simulink model "HILModelFull"  (Simulink 6.6)
settings: Solver=ode4  StartTime=0.0  StopTime=inf  FixedStep=SampleT  RelTol=1e-3
InitFcn:
  | clc
  | Taxi_Var_new
  | failures
  | insInit
  | piccolo_init
values from neighbouring files (symbols this model uses):
  A1 = 0    [Taxi_Var.m]
  Apolar = 0.0899    [Taxi_Var.m]
  CD0 = 0.0219    [Taxi_Var.m]
  chord = S/span    (= 0.384036716878)    [Taxi_Var.m]
  CL0 = 0.1857    [Taxi_Var.m]
  CLa = 4.6206    [Taxi_Var.m]
  CLa_dot = 1.93    [Taxi_Var.m]
  Clb = -0.0043    [Taxi_Var.m]
  ClDa = 0.1695    [Taxi_Var.m]
  CLDe = 0.4032    [Taxi_Var.m]
  CLDf = 0.047    [Taxi_Var.m]
  ClDr = 0.0003    [Taxi_Var.m]
  Clp = -0.4425    [Taxi_Var.m]
  CLq = 8.7465    [Taxi_Var.m]
  Clr = 0.0675    [Taxi_Var.m]
  Cm0 = -0.0902    [Taxi_Var.m]
  Cma = -1.3995    [Taxi_Var.m]
  CmDe = -0.9493    [Taxi_Var.m]
  CmDf = -.021    (= -0.021)    [Taxi_Var.m]
  Cmq = -10.8760    (= -10.876)    [Taxi_Var.m]
  Cnb = 0.0281    [Taxi_Var.m]
  CnDa = -0.0031    [Taxi_Var.m]
  CnDr = -0.0882    [Taxi_Var.m]
  Cnp = -0.0695    [Taxi_Var.m]
  Cnr = -0.1045    [Taxi_Var.m]
  CYb = -0.1999    [Taxi_Var.m]
  CYDr = 0.0192    [Taxi_Var.m]
  damax = 25*deg2rad    (= 0.436332312999)    [Taxi_Var.m]
  damin = -25*deg2rad    (= -0.436332312999)    [Taxi_Var.m]
  datrim = 0*deg2rad    (= 0)    [Taxi_Var.m]
  demax = 15*deg2rad    (= 0.261799387799)    [Taxi_Var.m]
  demin = -15*deg2rad    (= -0.261799387799)    [Taxi_Var.m]
  detrim = -2.4137*deg2rad    (= -0.0421270121554)    [Taxi_Var.m]
  dfland = 30*deg2rad    (= 0.523598775598)    [Taxi_Var.m]
  dfmax = 30*deg2rad    (= 0.523598775598)    [Taxi_Var.m]
  dfmin = 0*deg2rad    (= 0)    [Taxi_Var.m]
  drmax = 25*deg2rad    (= 0.436332312999)    [Taxi_Var.m]
  drmin = -25*deg2rad    (= -0.436332312999)    [Taxi_Var.m]
  drtrim = 0*deg2rad    (= 0)    [Taxi_Var.m]
  dtmax = 1    [Taxi_Var.m]
  dtmin = 0    [Taxi_Var.m]
  dttrim = 0.0725    [Taxi_Var.m]
  Euler_0 = [0; 0; 45]'*pi/180    [Taxi_Var.m]    (also in hilInit.m = [0; 0; 0*pi/180]')
  HIL_K = 3    [hilInit.m]    (also in insInit.m)
  ISA_g = 9.815    [Taxi_Var.m]
  ISA_hmax = 2000    [Taxi_Var.m]
  ISA_lapse = .0065    (= 0.0065)    [Taxi_Var.m]
  ISA_P0 = 101325    [Taxi_Var.m]
  ISA_R = 287    [Taxi_Var.m]
  ISA_rho0 = 1.225    [Taxi_Var.m]
  ISA_T0 = 289    [Taxi_Var.m]
  Ixx = 3.689084    [Taxi_Var.m]
  Iyy = 7.43789    [Taxi_Var.m]
  Izz = 10.22202    [Taxi_Var.m]
  mass = 22.5    [Taxi_Var.m]
  MinThK = 0.075    [Taxi_Var.m]
  Pos_0 = [0; 0; 1000]'    [Taxi_Var.m]    (also in hilInit.m = [500; 750; 350]')
  PQR_0 = [0; 0; 0]'    [Taxi_Var.m]
  span = 2.3368    [Taxi_Var.m]
  TFact = 0.4    [Taxi_Var.m]
  ThK = 2.18    [Taxi_Var.m]
  Vb_0 = [35; 0; 0]'    [Taxi_Var.m]
undefined symbols (not defined in the file or in its folder): clock, Earth, IdxCmdOrbitRadius, IdxCmdOrbitSense, IdxCmdWp1Alt, IdxCmdWp1Lat, IdxCmdWp1Lon, IdxCmdWp2Alt, IdxCmdWp2Lat, IdxCmdWp2Lon, IdxEstimReserved1, IdxEstimWEast, IdxEstimWNorth, IdxGainsAltD, IdxGainsAltI, IdxGainsAltP, IdxGainsPdynD, IdxGainsPdynI, IdxGainsPdynP, IdxGainsPitchD, IdxGainsPitchI, IdxGainsPitchP, IdxGainsRollD, IdxGainsRollI, IdxGainsRollP, IdxGainsSlopeElevatorD, IdxGainsSlopeElevatorP, IdxGainsTrackConv, IdxGainsTrackD, IdxGainsTrackI, IdxGainsTrackP, IdxGainsTurnD, IdxGainsTurnI, IdxGainsTurnP, IdxGainsYawD, IdxGainsYawI, IdxGainsYawP, IdxLimitsAileronMax, IdxLimitsAileronMin, IdxLimitsBankMax, IdxLimitsBankMin, IdxLimitsElevatorMax, IdxLimitsElevatorMin, IdxLimitsFlapMax, IdxLimitsFlapMin, IdxLimitsPdynMax, IdxLimitsPdynMin, IdxLimitsRudderMax, IdxLimitsRudderMin, IdxLimitsThrottleMax, IdxLimitsThrottleMin, IdxSensorsAlt, IdxSensorsLat, IdxSensorsLon, IdxSensorsVDown, IdxSensorsVEast, IdxSensorsVNorth, IdxStatesGlobal, IdxStatesManual, IdxStatesMode ... (+3)
libraries: piccolo_library x60, simulink x33, xpclib x8, aerolibasang x5, aerolibconvert2 x5, aerolibtransform2 x2, aerolibnav x2, aerolibatmos2 x1, dspmtrx3 x1
(part 2 of 4)

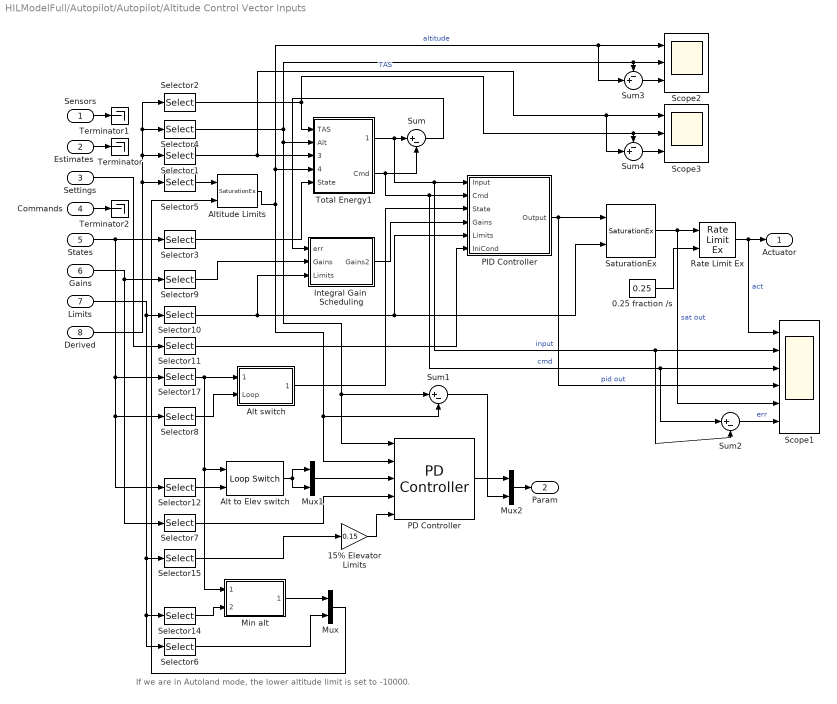
== system HILModelFull/Autopilot/Autopilot/Altitude Control Vector Inputs ==
  note: If we are in Autoland mode, the lower altitude limit is set to -10000.
  Sensors : Inport  PortDimensions=SizeSensors
  Estimates : Inport  Port=2  PortDimensions=SizeEstim
  Settings : Inport  Port=3  PortDimensions=SizeSet
  Commands : Inport  Port=4  PortDimensions=SizeCmd
  States : Inport  Port=5  PortDimensions=SizeStates
  Gains : Inport  Port=6  PortDimensions=SizeGains
  Limits : Inport  Port=7  PortDimensions=SizeLimits
  Derived : Inport  Port=8  PortDimensions=SizeDrv
  0.25 fraction /s : Constant  Value=0.25
  15% Elevator Limits : Gain  Gain=0.15  SaturateOnIntegerOverflow=on
  Alt switch : Subsystem  AncestorBlock=piccolo_library/Logic/DynP-Alt-Turn switch
  Alt to Elev switch : piccolo_library/Logic/Loop Switch  SystemSampleTime=-1
  Altitude Limits : piccolo_library/Nonlinear/SaturationEx  SystemSampleTime=-1
  Integral Gain  Scheduling : Subsystem
  Min alt : Subsystem
      mask Type: Loop Switch
      mask Description:
      | Select whether this individual loop is enabled or disabled.  This is done based on the specific
      | loop enable state, and the global flag.  In auto or manual steering the loop is on.  In Manual
      | or AutoLaunch the loop should be off.
  Mux : Mux  Inputs=2
  Mux1 : Mux  Inputs=2
  Mux2 : Mux  Inputs=2
  PD Controller : piccolo_library/Controllers/PD Controller  SystemSampleTime=-1  tsamp=tsamp  tdelay=0.5
  PID Controller : Subsystem  AncestorBlock=piccolo_library/Controllers/PID Controller  mask(PID Controller){tsamp=tsamp, tdelay=1}
      mask prompts: tsamp "Sample time:"; tdelay "Time derivative delay:"
      mask help: Generic PID (proportional, integral, derivative) controller with a single input and a single output.
  Rate Limit Ex : piccolo_library/Nonlinear/Rate Limit Ex  SystemSampleTime=-1  T=tsamp
  SaturationEx : piccolo_library/Nonlinear/SaturationEx  SystemSampleTime=-1
  Scope1 : Scope  NumInputPorts=6
      settings: YMin=0.120001~972.462~972.462~0.120001~0.120001~5.25e-006  YMax=0.120001~972.462~972.462~0.120001~0.120001~7e-006
  Scope2 : Scope  NumInputPorts=3
      settings: YMin=855~900.05~-0.475  YMax=945~900.475~-0.05  SaveName=ScopeData14
  Scope3 : Scope  NumInputPorts=3
      settings: YMin=35.0006~35~-0.035  YMax=35.0008~35.035~3.46945e-018  SaveName=ScopeData17
  Selector1 : Selector  IndexOptions=Index vector (dialog)  Indices=IdxDrvTASCmdNom  OutputSizes=1  InputPortWidth=SizeDrv
  Selector10 : Selector  IndexOptions=Index vector (dialog)  Indices=[IdxLimitsThrottleMin IdxLimitsThrottleMax]  OutputSizes=1  InputPortWidth=SizeLimits
  Selector11 : Selector  IndexOptions=Index vector (dialog)  Indices=IdxSetThrottleTrim  OutputSizes=1  InputPortWidth=SizeSet
  Selector12 : Selector  IndexOptions=Index vector (dialog)  Indices=IdxStatesAltToElev  OutputSizes=1  InputPortWidth=SizeStates
  Selector14 : Selector  IndexOptions=Index vector (dialog)  Indices=IdxLimitsAltMin  OutputSizes=1  InputPortWidth=SizeLimits
  Selector15 : Selector  IndexOptions=Index vector (dialog)  Indices=[IdxLimitsElevatorMin IdxLimitsElevatorMax]  OutputSizes=1  InputPortWidth=SizeLimits
  Selector17 : Selector  IndexOptions=Index vector (dialog)  Indices=[IdxStatesGlobal IdxStatesMode IdxStatesManual]  OutputSizes=1  InputPortWidth=SizeStates
  Selector2 : Selector  IndexOptions=Index vector (dialog)  Indices=IdxDrvTAS  OutputSizes=1  InputPortWidth=SizeDrv
  Selector3 : Selector  IndexOptions=Index vector (dialog)  Indices=IdxStatesPdyn  OutputSizes=1  InputPortWidth=SizeStates
  Selector4 : Selector  IndexOptions=Index vector (dialog)  Indices=IdxDrvBaroAlt  OutputSizes=1  InputPortWidth=SizeDrv
  Selector5 : Selector  IndexOptions=Index vector (dialog)  Indices=IdxDrvAltCmd  OutputSizes=1  InputPortWidth=SizeDrv
  Selector6 : Selector  IndexOptions=Index vector (dialog)  Indices=IdxLimitsAltMax  OutputSizes=1  InputPortWidth=SizeLimits
  Selector7 : Selector  IndexOptions=Index vector (dialog)  Indices=[IdxGainsSlopeElevatorP IdxGainsSlopeElevatorD]  OutputSizes=1  InputPortWidth=SizeGains
  Selector8 : Selector  IndexOptions=Index vector (dialog)  Indices=IdxStatesAlt  OutputSizes=1  InputPortWidth=SizeStates
  Selector9 : Selector  IndexOptions=Index vector (dialog)  Indices=[IdxGainsAltP IdxGainsAltI IdxGainsAltD]  OutputSizes=1  InputPortWidth=SizeGains
  Sum : Sum  Inputs=|+-  SaturateOnIntegerOverflow=on
  Sum1 : Sum  Inputs=|+-  SaturateOnIntegerOverflow=on
  Sum2 : Sum  Inputs=|+-  SaturateOnIntegerOverflow=on
  Sum3 : Sum  Inputs=-+|  SaturateOnIntegerOverflow=on
  Sum4 : Sum  Inputs=-+|  SaturateOnIntegerOverflow=on
  Terminator : Terminator
  Terminator1 : Terminator
  Terminator2 : Terminator
  Total Energy1 : Subsystem
      mask Type: Total Energy
      mask Description: Compute the total energy state and command as a sum of kinetic and potential energies, in units of altitude
  Actuator : Outport  OutDataType=fixdt(1,16,0)  OutScaling=[]
  Param : Outport  Port=2  OutDataType=fixdt(1,16,0)  OutScaling=[]
  wires:
  Total Energy1/2(Cmd) -> Sum/2, PID Controller/2(Cmd), Scope1/3, Sum2/1  "cmd"
  Total Energy1/1(Energy) -> Sum/1, PID Controller/1(Input), Scope1/2, Sum2/2  "input"
  Selector3/1 -> Total Energy1/5(State)
  Selector1/1 -> Total Energy1/3(TASCmd), Scope3/1, Sum4/2  "TAS"
  PD Controller/1 -> Mux2/1
  Mux2/1 -> Param/1
  Sum1/1 -> Mux2/2
  Commands/1 -> Terminator2/1
  States/1 -> Selector3/1, Selector12/1, Selector8/1, Selector17/1
  Sum/1 -> Integral Gain  Scheduling/1(err)
  Selector7/1 -> PD Controller/4
  Mux1/1 -> PD Controller/3
  Alt to Elev switch/1 -> Mux1/2, Mux1/1
  Selector15/1 -> 15% Elevator Limits/1
  15% Elevator Limits/1 -> PD Controller/5
  Selector9/1 -> Integral Gain  Scheduling/2(Gains)
  Integral Gain  Scheduling/1(Gains2) -> PID Controller/4(Gains)
  Mux/1 -> Altitude Limits/2
  Selector6/1 -> Mux/2
  Min alt/1(MinAltOut) -> Mux/1
  Selector14/1 -> Min alt/2(MinAlt)
  Selector12/1 -> Alt to Elev switch/2
  PID Controller/1(Output) -> SaturationEx/1, Scope1/4  "pid out"
  Derived/1 -> Selector1/1, Selector4/1, Selector2/1, Selector5/1
  Selector5/1 -> Altitude Limits/1
  Altitude Limits/1 -> Sum1/2, PD Controller/2, Total Energy1/4(AltCmd), Scope2/1, Sum3/2  "altitude"
  Selector4/1 -> Total Energy1/2(Alt), Sum1/1, PD Controller/1, Scope2/2, Sum3/1
  Selector2/1 -> Total Energy1/1(TAS), Scope3/2, Sum4/1
  Sensors/1 -> Terminator1/1
  Rate Limit Ex/1 -> Actuator/1, Scope1/1  "act"
  0.25 fraction /s/1 -> Rate Limit Ex/2
  SaturationEx/1 -> Rate Limit Ex/1, Scope1/5  "sat out"
  Selector10/1 -> Integral Gain  Scheduling/3(Limits), SaturationEx/2, PID Controller/5(Limits)
  Limits/1 -> Selector15/1, Selector6/1, Selector14/1, Selector10/1
  Gains/1 -> Selector7/1, Selector9/1
  Selector11/1 -> PID Controller/6(IniCond)
  Settings/1 -> Selector11/1
  Selector17/1 -> Alt switch/1(Globals), Min alt/1(Globals), Alt to Elev switch/1
  Selector8/1 -> Alt switch/2(Loop)
  Alt switch/1(TriOut) -> PID Controller/3(State)
  Estimates/1 -> Terminator/1
  Sum2/1 -> Scope1/6  "err"
  Sum3/1 -> Scope2/3
  Sum4/1 -> Scope3/3

== system HILModelFull/Autopilot/Autopilot/Flap Control Vector Inputs ==
  Sensors : Inport  PortDimensions=SizeSensors
  Estimates : Inport  Port=2  PortDimensions=SizeEstim
  Settings : Inport  Port=3  PortDimensions=SizeSet
  Commands : Inport  Port=4  PortDimensions=SizeCmd
  States : Inport  Port=5  PortDimensions=SizeStates
  Gains : Inport  Port=6  PortDimensions=SizeGains
  Limits : Inport  Port=7  PortDimensions=SizeLimits
  Derived : Inport  Port=8  PortDimensions=SizeDrv
  5 deg/s : Constant  Value=10*pi/180
  Direct Flap Control : Selector  IndexOptions=Index vector (dialog)  Indices=IdxCmdFlap  OutputSizes=1  InputPortWidth=SizeCmd
  Flap Loop Switch : piccolo_library/Logic/Loop Switch  SystemSampleTime=-1
  Landing Flap : Selector  IndexOptions=Index vector (dialog)  Indices=IdxSetLandingFlap  OutputSizes=1  InputPortWidth=SizeSet
  Rate Limit Ex : piccolo_library/Nonlinear/Rate Limit Ex  SystemSampleTime=-1  T=tsamp
  SaturationEx : piccolo_library/Nonlinear/SaturationEx  SystemSampleTime=-1
  Selector1 : Selector  IndexOptions=Index vector (dialog)  Indices=[IdxStatesGlobal IdxStatesMode IdxStatesManual]  OutputSizes=1  InputPortWidth=SizeStates
  Selector10 : Selector  IndexOptions=Index vector (dialog)  Indices=[IdxLimitsFlapMin IdxLimitsFlapMax]  OutputSizes=1  InputPortWidth=SizeLimits
  Selector12 : Selector  IndexOptions=Index vector (dialog)  Indices=IdxStatesSlope  OutputSizes=1  InputPortWidth=SizeStates
  Selector2 : Selector  IndexOptions=Index vector (dialog)  Indices=IdxStatesFlap  OutputSizes=1  InputPortWidth=SizeStates
  Switch : Switch  Threshold=0.5  SaturateOnIntegerOverflow=on
  Switch1 : Switch  Threshold=0.5  SaturateOnIntegerOverflow=on
  Terminator{1..4} (4 alike) : Terminator
  Zero : Constant  Value=0
  Actuator : Outport  OutDataType=fixdt(1,16,0)  OutScaling=[]
  wires:
  Sensors/1 -> Terminator1/1
  Selector10/1 -> SaturationEx/2
  Selector12/1 -> Switch/2
  Direct Flap Control/1 -> Switch/3
  Landing Flap/1 -> Switch/1
  Estimates/1 -> Terminator2/1
  Gains/1 -> Terminator3/1
  Derived/1 -> Terminator4/1
  Settings/1 -> Landing Flap/1
  Commands/1 -> Direct Flap Control/1
  States/1 -> Selector12/1, Selector2/1, Selector1/1
  Limits/1 -> Selector10/1
  Switch/1 -> Switch1/1
  Flap Loop Switch/1 -> Switch1/2
  Switch1/1 -> SaturationEx/1
  Selector1/1 -> Flap Loop Switch/1
  Selector2/1 -> Flap Loop Switch/2
  Zero/1 -> Switch1/3
  SaturationEx/1 -> Rate Limit Ex/1
  Rate Limit Ex/1 -> Actuator/1
  5 deg/s/1 -> Rate Limit Ex/2

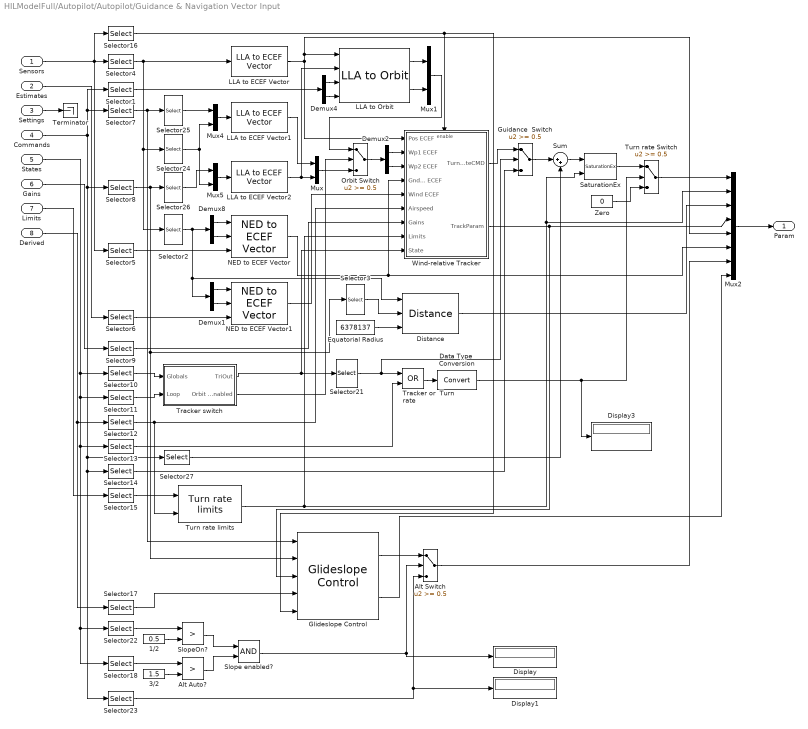
== system HILModelFull/Autopilot/Autopilot/Guidance & Navigation Vector Input ==
  Sensors : Inport  PortDimensions=SizeSensors
  Estimates : Inport  Port=2  PortDimensions=SizeEstim
  Settings : Inport  Port=3  PortDimensions=SizeSet
  Commands : Inport  Port=4  PortDimensions=SizeCmd
  States : Inport  Port=5  PortDimensions=SizeStates
  Gains : Inport  Port=6  PortDimensions=SizeGains
  Limits : Inport  Port=7  PortDimensions=SizeLimits
  Derived : Inport  Port=8  PortDimensions=SizeDrv
  1/2 : Constant  Value=0.5
  3/2 : Constant  Value=1.5
  Alt Auto? : RelationalOperator  Operator=>
  Alt Switch : Switch  Threshold=0.5  SaturateOnIntegerOverflow=on
  Data Type  Conversion : DataTypeConversion  OutDataTypeMode=double  OutDataType=fixdt(1,16,0)  OutScaling=[]  SaturateOnIntegerOverflow=on  RndMeth=Zero
  Demux{1..2,4,8} (4 alike) : Demux  Outputs=2
  Display : Display
  Display1 : Display
  Display3 : Display
  Distance : piccolo_library/Transformations/Distance  SystemSampleTime=-1
  Equatorial Radius : Constant  Value=6378137
  Glideslope Control : piccolo_library/Controllers/Guidance/Glideslope Control  SystemSampleTime=-1  tsamp=tsamp  aptsamp=aptsamp
  Guidance  Switch : Switch  Threshold=0.5  SaturateOnIntegerOverflow=on
  LLA to ECEF Vector : piccolo_library/Transformations/LLA to ECEF Vector  SystemSampleTime=-1
  LLA to ECEF Vector1 : piccolo_library/Transformations/LLA to ECEF Vector  SystemSampleTime=-1
  LLA to ECEF Vector2 : piccolo_library/Transformations/LLA to ECEF Vector  SystemSampleTime=-1
  LLA to Orbit : piccolo_library/Controllers/Guidance/LLA to Orbit  SystemSampleTime=-1
  Mux{,1,4..5} (4 alike) : Mux  Inputs=2
  Mux2 : Mux  Inputs=[1 2 1 5 3 3 1 3]
  NED to ECEF Vector : piccolo_library/Transformations/NED to ECEF Vector  SystemSampleTime=-1
  NED to ECEF Vector1 : piccolo_library/Transformations/NED to ECEF Vector  SystemSampleTime=-1
  Orbit Switch : Switch  Threshold=0.5  SaturateOnIntegerOverflow=on
  SaturationEx : piccolo_library/Nonlinear/SaturationEx  SystemSampleTime=-1
  Selector1 : Selector  IndexOptions=Index vector (dialog)  Indices=[IdxCmdOrbitRadius IdxCmdOrbitSense]  OutputSizes=1  InputPortWidth=SizeCmd
  Selector10 : Selector  IndexOptions=Index vector (dialog)  Indices=[IdxStatesGlobal IdxStatesMode IdxStatesManual]  OutputSizes=1  InputPortWidth=SizeStates
  Selector11 : Selector  IndexOptions=Index vector (dialog)  Indices=IdxStatesTracker  OutputSizes=1  InputPortWidth=SizeStates
  Selector12 : Selector  IndexOptions=Index vector (dialog)  Indices=IdxDrvTAS  OutputSizes=1  InputPortWidth=SizeDrv
  Selector13 : Selector  IndexOptions=Index vector (dialog)  Indices=IdxStatesTurnRate  OutputSizes=1  InputPortWidth=SizeStates
  Selector14 : Selector  IndexOptions=Index vector (dialog)  Indices=IdxCmdTurnRate  OutputSizes=1  InputPortWidth=SizeCmd
  Selector15 : Selector  IndexOptions=Index vector (dialog)  Indices=[IdxLimitsBankMin IdxLimitsBankMax]  OutputSizes=1  InputPortWidth=SizeLimits
  Selector16 : Selector  IndexOptions=Index vector (dialog)  Indices=IdxSensorsGPSNew  OutputSizes=1  InputPortWidth=SizeSensors
  Selector17 : Selector  IndexOptions=Index vector (dialog)  Indices=IdxDrvBaroAlt  OutputSizes=1  InputPortWidth=SizeDrv
  Selector18 : Selector  IndexOptions=Index vector (dialog)  Indices=IdxStatesAlt  OutputSizes=1  InputPortWidth=SizeStates
  Selector{2..3,25..26} (4 alike) : Selector  IndexOptions=Index vector (dialog)  Indices=[1 2]  OutputSizes=1  InputPortWidth=3
  Selector21 : Selector  IndexOptions=Index vector (dialog)  Indices=2  OutputSizes=1  InputPortWidth=3
  Selector22 : Selector  IndexOptions=Index vector (dialog)  Indices=IdxStatesSlope  OutputSizes=1  InputPortWidth=SizeStates
  Selector23 : Selector  IndexOptions=Index vector (dialog)  Indices=IdxCmdAlt  OutputSizes=1  InputPortWidth=SizeCmd
  Selector24 : Selector  IndexOptions=Index vector (dialog)  Indices=3  OutputSizes=1  InputPortWidth=3
  Selector27 : Selector  IndexOptions=Index vector (dialog)  Indices=IdxCmdTurnRateShift  OutputSizes=1  InputPortWidth=SizeCmd
  Selector4 : Selector  IndexOptions=Index vector (dialog)  Indices=[IdxSensorsLat IdxSensorsLon IdxSensorsAlt]  OutputSizes=1  InputPortWidth=SizeSensors
  Selector5 : Selector  IndexOptions=Index vector (dialog)  Indices=[IdxSensorsVNorth IdxSensorsVEast IdxSensorsVDown]  OutputSizes=1  InputPortWidth=SizeSensors
  Selector6 : Selector  IndexOptions=Index vector (dialog)  Indices=[IdxEstimWNorth IdxEstimWEast IdxEstimReserved1]  OutputSizes=1  InputPortWidth=SizeEstim
  Selector7 : Selector  IndexOptions=Index vector (dialog)  Indices=[IdxCmdWp1Lat IdxCmdWp1Lon IdxCmdWp1Alt]  OutputSizes=1  InputPortWidth=SizeCmd
  Selector8 : Selector  IndexOptions=Index vector (dialog)  Indices=[IdxCmdWp2Lat IdxCmdWp2Lon IdxCmdWp2Alt]  OutputSizes=1  InputPortWidth=SizeCmd
  Selector9 : Selector  IndexOptions=Index vector (dialog)  Indices=[IdxGainsTrackP IdxGainsTrackI IdxGainsTrackD IdxGainsTrackConv]  OutputSizes=1  InputPortWidth=SizeGains
  Slope enabled? : Logic  AllPortsSameDT=off
  SlopeOn? : RelationalOperator  Operator=>
  Sum : Sum  Inputs=|++  SaturateOnIntegerOverflow=on
  Terminator : Terminator
  Tracker or  Turn rate : Logic  Operator=OR  AllPortsSameDT=off
  Tracker switch : Subsystem  AncestorBlock=piccolo_library/Logic/Tracker switch
  Turn rate Switch : Switch  Threshold=0.5  SaturateOnIntegerOverflow=on
  Turn rate limits : piccolo_library/Flight Mechanics/Turn rate limits  SystemSampleTime=-1
  Wind-relative Tracker : Subsystem  AncestorBlock=piccolo_library/Controllers/Guidance/Wind-relative Tracker  mask(Wind-relative Tracker){tsamp=tsamp}
      mask prompts: tsamp "Sample time:"
      mask help: A lateral track control law that takes into account the wind speed.
  Zero : Constant  Value=0
  Param : Outport  OutDataType=fixdt(1,16,0)  OutScaling=[]
  wires:
  Slope enabled?/1 -> Alt Switch/2, Display/1
  Alt Auto?/1 -> Slope enabled?/2
  SlopeOn?/1 -> Slope enabled?/1
  3/2/1 -> Alt Auto?/2
  Selector18/1 -> Alt Auto?/1
  Selector22/1 -> SlopeOn?/1
  1/2/1 -> SlopeOn?/2
  Selector21/1 -> Tracker or  Turn rate/1, Guidance  Switch/2
  Selector27/1 -> Sum/2
  Sum/1 -> SaturationEx/1
  Guidance  Switch/1 -> Sum/1
  Glideslope Control/2 -> Mux2/8
  Glideslope Control/1 -> Alt Switch/1
  Selector17/1 -> Glideslope Control/4
  Selector26/1 -> Mux5/1
  Selector7/1 -> Glideslope Control/1, Selector25/1
  Selector25/1 -> Mux4/1
  Selector24/1 -> Mux5/2, Mux4/2
  Mux5/1 -> LLA to ECEF Vector2/1
  Mux4/1 -> LLA to ECEF Vector1/1
  Alt Switch/1 -> Mux2/7
  Selector23/1 -> Alt Switch/3, Display1/1
  LLA to Orbit/2 -> Mux1/2
  LLA to Orbit/1 -> Mux1/1
  Selector1/1 -> Demux4/1
  Demux4/2 -> LLA to Orbit/4
  Demux4/1 -> LLA to Orbit/3
  Selector16/1 -> Glideslope Control/5, Wind-relative Tracker/Enable
  Settings/1 -> Terminator/1
  Data Type  Conversion/1 -> Turn rate Switch/2, Display3/1
  Wind-relative Tracker/2(TrackParam) -> Glideslope Control/3, Mux2/4
  Distance/1 -> Mux2/3
  Zero/1 -> Turn rate Switch/3
  SaturationEx/1 -> Turn rate Switch/1
  Tracker or  Turn rate/1 -> Data Type  Conversion/1
  Selector13/1 -> Tracker or  Turn rate/2
  Turn rate limits/1 -> Mux2/2, SaturationEx/2, Wind-relative Tracker/8(Limits)
  Limits/1 -> Selector15/1
  Selector15/1 -> Turn rate limits/1
  Selector14/1 -> Guidance  Switch/3
  Wind-relative Tracker/1(TurnRateCMD) -> Guidance  Switch/1
  Mux2/1 -> Param/1
  Tracker switch/1(TriOut) -> Wind-relative Tracker/9(State), Selector21/1
  Tracker switch/2(Orbit Enabled) -> Orbit Switch/2
  Selector11/1 -> Tracker switch/2(Loop)
  Selector10/1 -> Tracker switch/1(Globals)
  Derived/1 -> Selector17/1, Selector12/1
  States/1 -> Selector18/1, Selector22/1, Selector13/1, Selector11/1, Selector10/1
  Gains/1 -> Selector9/1
  Commands/1 -> Selector1/1, Selector7/1, Selector27/1, Selector23/1, Selector14/1, Selector8/1
  Selector8/1 -> Glideslope Control/2, Selector3/1, Selector26/1
  Estimates/1 -> Selector6/1
  Selector5/1 -> NED to ECEF Vector/3
  Sensors/1 -> Selector16/1, Selector5/1, Selector4/1
  Selector4/1 -> Selector2/1, Selector24/1, LLA to ECEF Vector/1
  Demux8/1 -> NED to ECEF Vector/1
  Demux8/2 -> NED to ECEF Vector/2
  Selector2/1 -> Demux8/1, Demux1/1, Distance/1
  Demux1/1 -> NED to ECEF Vector1/1
  Demux1/2 -> NED to ECEF Vector1/2
  Selector6/1 -> NED to ECEF Vector1/3
  LLA to ECEF Vector/1 -> LLA to Orbit/1, Mux2/5, Wind-relative Tracker/1(Pos ECEF)
  LLA to ECEF Vector2/1 -> LLA to Orbit/2, Mux/2
  Selector9/1 -> Wind-relative Tracker/7(Gains)
  LLA to ECEF Vector1/1 -> Mux/1
  Mux/1 -> Orbit Switch/3
  Mux1/1 -> Orbit Switch/1
  Demux2/1 -> Wind-relative Tracker/2(Wp1 ECEF)
  Demux2/2 -> Wind-relative Tracker/3(Wp2 ECEF)
  Orbit Switch/1 -> Demux2/1
  NED to ECEF Vector/1 -> Mux2/6, Wind-relative Tracker/4(Gndspd ECEF)
  NED to ECEF Vector1/1 -> Wind-relative Tracker/5(Wind ECEF)
  Selector12/1 -> Turn rate limits/2, Wind-relative Tracker/6(Airspeed)
  Equatorial Radius/1 -> Distance/3
  Selector3/1 -> Distance/2
  Turn rate Switch/1 -> Mux2/1

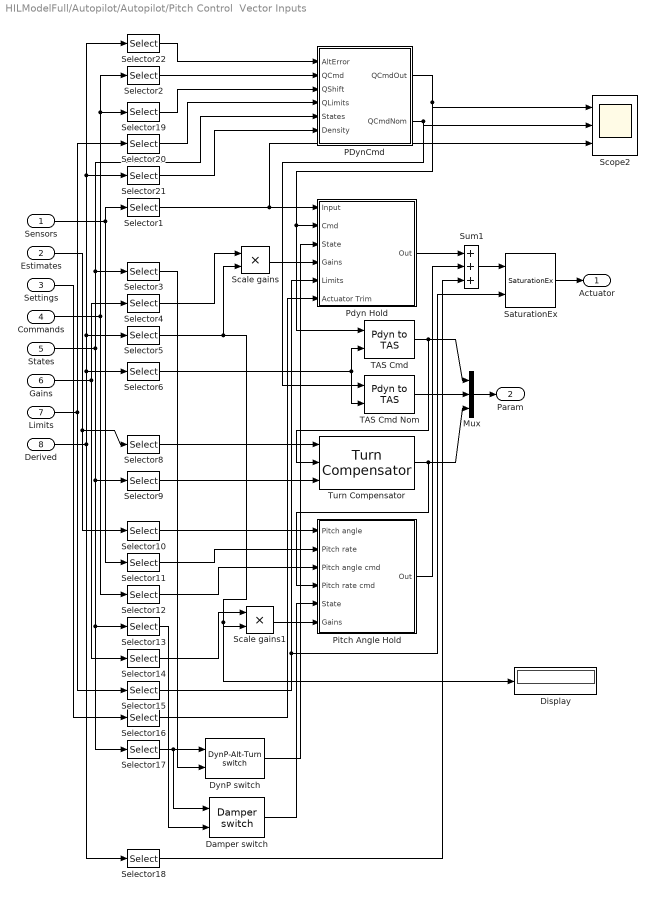
== system HILModelFull/Autopilot/Autopilot/Pitch Control  Vector Inputs ==
  Sensors : Inport  PortDimensions=SizeSensors
  Estimates : Inport  Port=2  PortDimensions=SizeEstim
  Settings : Inport  Port=3  PortDimensions=SizeSet
  Commands : Inport  Port=4  PortDimensions=SizeCmd
  States : Inport  Port=5  PortDimensions=SizeStates
  Gains : Inport  Port=6  PortDimensions=SizeGains
  Limits : Inport  Port=7  PortDimensions=SizeLimits
  Derived : Inport  Port=8  PortDimensions=SizeDrv
  Damper switch : piccolo_library/Logic/Damper switch  SystemSampleTime=-1
  Display : Display
  DynP switch : piccolo_library/Logic/DynP-Alt-Turn switch  SystemSampleTime=-1
  Mux : Mux  Inputs=3
  PDynCmd : Subsystem
  Pdyn Hold : Subsystem  AncestorBlock=piccolo_library/Controllers/Longitudinal/Pdyn Hold  mask(Dynamic pressure hold){tsamp=tsamp}
      mask prompts: tsamp "Sample time:"
      mask help: Control the dynamic pressure using elevator command.
  Pitch Angle Hold : Subsystem  AncestorBlock=piccolo_library/Controllers/Longitudinal/Pitch Angle Hold  mask(Pitch angle hold){tsamp=tsamp}
      mask prompts: tsamp "Sample time:"
      mask help: Pitch angle hold with proportional and derivative terms.
  SaturationEx : piccolo_library/Nonlinear/SaturationEx  SystemSampleTime=-1
  Scale gains : Product  SaturateOnIntegerOverflow=on  InputSameDT=on
  Scale gains1 : Product  SaturateOnIntegerOverflow=on  InputSameDT=on
  Scope2 : Scope  NumInputPorts=3
      settings: YMin=687.696~687.696~688.4  YMax=687.696~687.696~688.775  SaveName=ScopeData3
  Selector1 : Selector  IndexOptions=Index vector (dialog)  Indices=IdxSensorsPdyn  OutputSizes=1  InputPortWidth=SizeSensors
  Selector10 : Selector  IndexOptions=Index vector (dialog)  Indices=IdxEstimPitchAngle  OutputSizes=1  InputPortWidth=SizeEstim
  Selector11 : Selector  IndexOptions=Index vector (dialog)  Indices=IdxSensorsPitchRate  OutputSizes=1  InputPortWidth=SizeSensors
  Selector12 : Selector  IndexOptions=Index vector (dialog)  Indices=IdxCmdPitchAngle  OutputSizes=1  InputPortWidth=SizeCmd
  Selector13 : Selector  IndexOptions=Index vector (dialog)  Indices=IdxStatesPitch  OutputSizes=1  InputPortWidth=SizeStates
  Selector14 : Selector  IndexOptions=Index vector (dialog)  Indices=[IdxGainsPitchP IdxGainsPitchI IdxGainsPitchD]  OutputSizes=1  InputPortWidth=SizeGains
  Selector15 : Selector  IndexOptions=Index vector (dialog)  Indices=[IdxLimitsElevatorMin IdxLimitsElevatorMax]  OutputSizes=1  InputPortWidth=SizeLimits
  Selector16 : Selector  IndexOptions=Index vector (dialog)  Indices=IdxSetElevatorTrim  OutputSizes=1  InputPortWidth=SizeSet
  Selector17 : Selector  IndexOptions=Index vector (dialog)  Indices=[IdxStatesGlobal IdxStatesMode IdxStatesManual]  OutputSizes=1  InputPortWidth=SizeStates
  Selector18 : Selector  IndexOptions=Index vector (dialog)  Indices=IdxDrvSlopeElevator  OutputSizes=1  InputPortWidth=SizeDrv
  Selector19 : Selector  IndexOptions=Index vector (dialog)  Indices=IdxCmdPdynShift  OutputSizes=1  InputPortWidth=SizeCmd
  Selector2 : Selector  IndexOptions=Index vector (dialog)  Indices=IdxCmdPdyn  OutputSizes=1  InputPortWidth=SizeCmd
  Selector20 : Selector  IndexOptions=Index vector (dialog)  Indices=[IdxLimitsPdynMin IdxLimitsPdynMax]  OutputSizes=1  InputPortWidth=SizeLimits
  Selector21 : Selector  IndexOptions=Index vector (dialog)  Indices=IdxDrvDensity  OutputSizes=1  InputPortWidth=SizeDrv
  Selector22 : Selector  IndexOptions=Index vector (dialog)  Indices=IdxDrvAltError  OutputSizes=1  InputPortWidth=SizeDrv
  Selector3 : Selector  IndexOptions=Index vector (dialog)  Indices=IdxStatesPdyn  OutputSizes=1  InputPortWidth=SizeStates
  Selector4 : Selector  IndexOptions=Index vector (dialog)  Indices=[IdxGainsPdynP IdxGainsPdynI IdxGainsPdynD]  OutputSizes=1  InputPortWidth=SizeGains
  Selector5 : Selector  IndexOptions=Index vector (dialog)  Indices=IdxDrvGainScaler  OutputSizes=1  InputPortWidth=SizeDrv
  Selector6 : Selector  IndexOptions=Index vector (dialog)  Indices=IdxDrvDensity  OutputSizes=1  InputPortWidth=SizeDrv
  Selector8 : Selector  IndexOptions=Index vector (dialog)  Indices=IdxEstimRollAngle  OutputSizes=1  InputPortWidth=SizeEstim
  Selector9 : Selector  IndexOptions=Index vector (dialog)  Indices=IdxStatesTurnComp  OutputSizes=1  InputPortWidth=SizeStates
  Sum1 : Sum  Inputs=+++  SaturateOnIntegerOverflow=on  InputSameDT=on
  TAS Cmd : piccolo_library/Flight Mechanics/Pdyn to TAS  SystemSampleTime=-1
  TAS Cmd Nom : piccolo_library/Flight Mechanics/Pdyn to TAS  SystemSampleTime=-1
  Turn Compensator : piccolo_library/Controllers/Longitudinal/Turn Compensator  SystemSampleTime=-1
  Actuator : Outport  OutDataType=fixdt(1,16,0)  OutScaling=[]
  Param : Outport  Port=2  OutDataType=fixdt(1,16,0)  OutScaling=[]
  wires:
  PDynCmd/2(QCmdNom) -> TAS Cmd Nom/1, Scope2/2
  TAS Cmd Nom/1 -> Mux/2
  PDynCmd/1(QCmdOut) -> TAS Cmd/1, Pdyn Hold/2(Cmd), Scope2/1
  Selector22/1 -> PDynCmd/1(AltError)
  Selector21/1 -> PDynCmd/6(Density)
  Selector20/1 -> PDynCmd/4(QLimits)
  Selector19/1 -> PDynCmd/3(QShift)
  Selector2/1 -> PDynCmd/2(QCmd)
  Damper switch/1 -> Pitch Angle Hold/5(State)
  DynP switch/1 -> Pdyn Hold/3(State)
  Selector9/1 -> Turn Compensator/3
  Selector18/1 -> Sum1/3
  Selector13/1 -> Damper switch/2
  Selector3/1 -> DynP switch/2
  Selector17/1 -> Damper switch/1, DynP switch/1
  Mux/1 -> Param/1
  Settings/1 -> Selector16/1
  Selector16/1 -> Pdyn Hold/6(Actuator Trim)
  Estimates/1 -> Selector8/1, Selector10/1
  Limits/1 -> Selector20/1, Selector15/1
  Derived/1 -> Selector18/1, Selector22/1, Selector21/1, Selector5/1, Selector6/1
  Gains/1 -> Selector14/1, Selector4/1
  States/1 -> PDynCmd/5(States), Selector3/1, Selector17/1, Selector13/1, Selector9/1
  Commands/1 -> Selector19/1, Selector2/1, Selector12/1
  Sensors/1 -> Selector11/1, Selector1/1
  Selector1/1 -> Pdyn Hold/1(Input), Scope2/3
  TAS Cmd/1 -> Mux/1, Turn Compensator/2
  Selector8/1 -> Turn Compensator/1
  Selector10/1 -> Pitch Angle Hold/1(Pitch angle)
  Selector11/1 -> Pitch Angle Hold/2(Pitch rate)
  Turn Compensator/1 -> Mux/3, Pitch Angle Hold/4(Pitch rate cmd)
  Selector12/1 -> Pitch Angle Hold/3(Pitch angle cmd)
  Scale gains/1 -> Pdyn Hold/4(Gains)
  Selector4/1 -> Scale gains/1
  Selector5/1 -> Scale gains/2, Scale gains1/2, Display/1
  Selector6/1 -> TAS Cmd Nom/2, TAS Cmd/2
  Scale gains1/1 -> Pitch Angle Hold/6(Gains)
  Selector14/1 -> Scale gains1/1
  Selector15/1 -> Pdyn Hold/5(Limits), SaturationEx/2
  Pdyn Hold/1(Out) -> Sum1/1
  Pitch Angle Hold/1(Out) -> Sum1/2
  Sum1/1 -> SaturationEx/1
  SaturationEx/1 -> Actuator/1

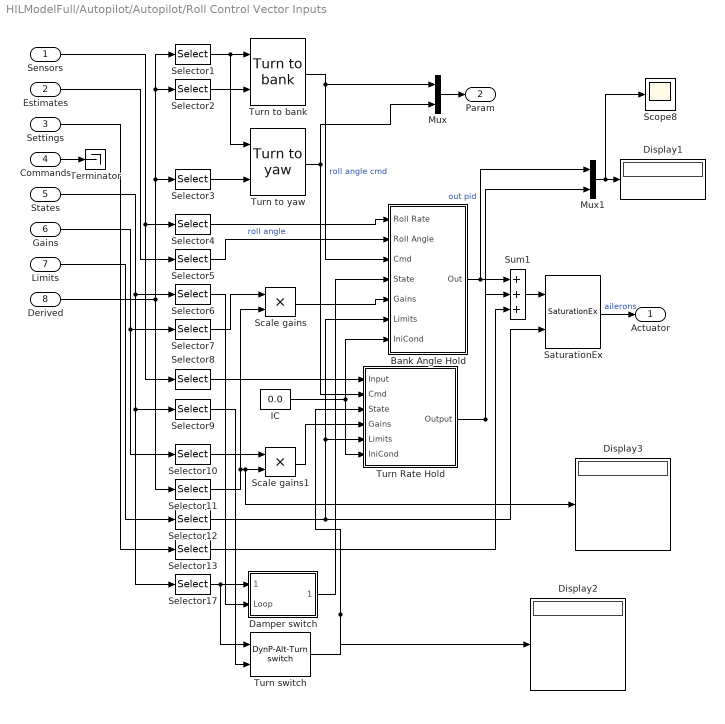
== system HILModelFull/Autopilot/Autopilot/Roll Control Vector Inputs ==
  Sensors : Inport  PortDimensions=SizeSensors
  Estimates : Inport  Port=2  PortDimensions=SizeEstim
  Settings : Inport  Port=3  PortDimensions=SizeSet
  Commands : Inport  Port=4  PortDimensions=SizeCmd
  States : Inport  Port=5  PortDimensions=SizeStates
  Gains : Inport  Port=6  PortDimensions=SizeGains
  Limits : Inport  Port=7  PortDimensions=SizeLimits
  Derived : Inport  Port=8  PortDimensions=SizeDrv
  Bank Angle Hold : Subsystem  AncestorBlock=piccolo_library/Controllers/Lateral/Bank Angle Hold
  Damper switch : Subsystem  AncestorBlock=piccolo_library/Logic/Damper switch
  Display1 : Display
  Display2 : Display
  Display3 : Display
  IC : Constant  Value=0.0
  Mux : Mux  Inputs=2
  Mux1 : Mux  Inputs=2
  SaturationEx : piccolo_library/Nonlinear/SaturationEx  SystemSampleTime=-1
  Scale gains : Product  SaturateOnIntegerOverflow=on  InputSameDT=on
  Scale gains1 : Product  SaturateOnIntegerOverflow=on  InputSameDT=on
  Scope8 : Scope
      settings: YMin=-0.6  YMax=0.6  SaveName=ScopeData26
  Selector1 : Selector  IndexOptions=Index vector (dialog)  Indices=IdxDrvTurnRateCmd  OutputSizes=1  InputPortWidth=SizeDrv
  Selector10 : Selector  IndexOptions=Index vector (dialog)  Indices=[IdxGainsTurnP IdxGainsTurnI IdxGainsTurnD]  OutputSizes=1  InputPortWidth=SizeGains
  Selector11 : Selector  IndexOptions=Index vector (dialog)  Indices=IdxDrvGainScaler  OutputSizes=1  InputPortWidth=SizeDrv
  Selector12 : Selector  IndexOptions=Index vector (dialog)  Indices=[IdxLimitsAileronMin IdxLimitsAileronMax]  OutputSizes=1  InputPortWidth=SizeLimits
  Selector13 : Selector  IndexOptions=Index vector (dialog)  Indices=IdxSetAileronTrim  OutputSizes=1  InputPortWidth=SizeSet
  Selector17 : Selector  IndexOptions=Index vector (dialog)  Indices=[IdxStatesGlobal IdxStatesMode IdxStatesManual]  OutputSizes=1  InputPortWidth=SizeStates
  Selector2 : Selector  IndexOptions=Index vector (dialog)  Indices=IdxDrvTAS  OutputSizes=1  InputPortWidth=SizeDrv
  Selector3 : Selector  IndexOptions=Index vector (dialog)  Indices=IdxDrvTAS  OutputSizes=1  InputPortWidth=SizeDrv
  Selector4 : Selector  IndexOptions=Index vector (dialog)  Indices=IdxSensorsRollRate  OutputSizes=1  InputPortWidth=SizeSensors
  Selector5 : Selector  IndexOptions=Index vector (dialog)  Indices=IdxEstimRollAngle  OutputSizes=1  InputPortWidth=SizeEstim
  Selector6 : Selector  IndexOptions=Index vector (dialog)  Indices=IdxStatesRoll  OutputSizes=1  InputPortWidth=SizeStates
  Selector7 : Selector  IndexOptions=Index vector (dialog)  Indices=[IdxGainsRollP IdxGainsRollI IdxGainsRollD]  OutputSizes=1  InputPortWidth=SizeGains
  Selector8 : Selector  IndexOptions=Index vector (dialog)  Indices=IdxSensorsYawRate  OutputSizes=1  InputPortWidth=SizeSensors
  Selector9 : Selector  IndexOptions=Index vector (dialog)  Indices=IdxStatesTurnRate  OutputSizes=1  InputPortWidth=SizeStates
  Sum1 : Sum  Inputs=+++  SaturateOnIntegerOverflow=on  InputSameDT=on
  Terminator : Terminator
  Turn Rate Hold : Subsystem  AncestorBlock=piccolo_library/Controllers/PID Controller  mask(PID Controller){tsamp=tsamp, tdelay=0.25}
      mask prompts: tsamp "Sample time:"; tdelay "Time derivative delay:"
      mask help: Generic PID (proportional, integral, derivative) controller with a single input and a single output.
  Turn switch : piccolo_library/Logic/DynP-Alt-Turn switch  SystemSampleTime=-1
  Turn to bank : piccolo_library/Flight Mechanics/Turn to bank  SystemSampleTime=-1
  Turn to yaw : piccolo_library/Flight Mechanics/Turn to yaw  SystemSampleTime=-1
  Actuator : Outport  OutDataType=fixdt(1,16,0)  OutScaling=[]
  Param : Outport  Port=2  OutDataType=fixdt(1,16,0)  OutScaling=[]
  wires:
  IC/1 -> Turn Rate Hold/6(IniCond), Bank Angle Hold/7(IniCond)
  Commands/1 -> Terminator/1
  Turn switch/1 -> Turn Rate Hold/3(State), Display2/1
  Selector9/1 -> Turn switch/2
  Damper switch/1(TriOut) -> Bank Angle Hold/4(State)
  Selector6/1 -> Damper switch/2(Loop)
  Selector17/1 -> Damper switch/1(Globals), Turn switch/1
  Mux/1 -> Param/1
  Settings/1 -> Selector13/1
  Selector13/1 -> Sum1/3
  Limits/1 -> Selector12/1
  Gains/1 -> Selector10/1, Selector7/1
  States/1 -> Selector17/1, Selector9/1, Selector6/1
  Estimates/1 -> Selector5/1
  Sensors/1 -> Selector8/1, Selector4/1
  Derived/1 -> Selector11/1, Selector1/1, Selector2/1, Selector3/1
  SaturationEx/1 -> Actuator/1  "ailerons"
  Sum1/1 -> SaturationEx/1
  Turn Rate Hold/1(Output) -> Sum1/2, Mux1/2
  Bank Angle Hold/1(Out) -> Sum1/1, Mux1/1  "out pid"
  Selector12/1 -> SaturationEx/2, Turn Rate Hold/5(Limits), Bank Angle Hold/6(Limits)
  Selector11/1 -> Scale gains/2, Scale gains1/2, Display3/1
  Selector10/1 -> Scale gains1/1
  Scale gains1/1 -> Turn Rate Hold/4(Gains)
  Selector7/1 -> Scale gains/1
  Scale gains/1 -> Bank Angle Hold/5(Gains)
  Turn to yaw/1 -> Mux/2, Turn Rate Hold/2(Cmd)
  Selector8/1 -> Turn Rate Hold/1(Input)
  Turn to bank/1 -> Mux/1, Bank Angle Hold/3(Cmd)  "roll angle cmd"
  Selector5/1 -> Bank Angle Hold/2(Roll Angle)  "roll angle"
  Selector4/1 -> Bank Angle Hold/1(Roll Rate)
  Selector3/1 -> Turn to yaw/2
  Selector2/1 -> Turn to bank/2
  Selector1/1 -> Turn to yaw/1, Turn to bank/1
  Mux1/1 -> Display1/1, Scope8/1

== system HILModelFull/Autopilot/Autopilot/Yaw Control Vector Inputs ==
  note: Yaw integral
      | must be zero
  Sensors : Inport  PortDimensions=SizeSensors
  Estimates : Inport  Port=2  PortDimensions=SizeEstim
  Settings : Inport  Port=3  PortDimensions=SizeSet
  Commands : Inport  Port=4  PortDimensions=SizeCmd
  States : Inport  Port=5  PortDimensions=SizeStates
  Gains : Inport  Port=6  PortDimensions=SizeGains
  Limits : Inport  Port=7  PortDimensions=SizeLimits
  Derived : Inport  Port=8  PortDimensions=SizeDrv
  Demux : Demux  Outputs=3
  Initial condition : Constant  Value=0.0
  Mux : Mux  Inputs=3
  SaturationEx : piccolo_library/Nonlinear/SaturationEx  SystemSampleTime=-1
  Scale gains : Product  SaturateOnIntegerOverflow=on  InputSameDT=on
  Scope : Scope  NumInputPorts=3
      settings: YMin=-1~-0.015~-0.015  YMax=1~0.015~0.015  SaveName=ScopeData22
  Selector1 : Selector  IndexOptions=Index vector (dialog)  Indices=IdxSensorsYawRate  OutputSizes=1  InputPortWidth=SizeSensors
  Selector17 : Selector  IndexOptions=Index vector (dialog)  Indices=[IdxStatesGlobal IdxStatesMode IdxStatesManual]  OutputSizes=1  InputPortWidth=SizeStates
  Selector2 : Selector  IndexOptions=Index vector (dialog)  Indices=IdxDrvTurnRateCmd  OutputSizes=1  InputPortWidth=SizeDrv
  Selector3 : Selector  IndexOptions=Index vector (dialog)  Indices=IdxStatesYaw  OutputSizes=1  InputPortWidth=SizeStates
  Selector4 : Selector  IndexOptions=Index vector (dialog)  Indices=[IdxGainsYawP IdxGainsYawI IdxGainsYawD]  OutputSizes=1  InputPortWidth=SizeGains
  Selector5 : Selector  IndexOptions=Index vector (dialog)  Indices=IdxDrvGainScaler  OutputSizes=1  InputPortWidth=SizeDrv
  Selector6 : Selector  IndexOptions=Index vector (dialog)  Indices=[IdxLimitsRudderMin IdxLimitsRudderMax]  OutputSizes=1  InputPortWidth=SizeLimits
  Selector7 : Selector  IndexOptions=Index vector (dialog)  Indices=IdxSetRudderTrim  OutputSizes=1  InputPortWidth=SizeSet
  Selector8 : Selector  IndexOptions=Index vector (dialog)  Indices=IdxDrvTAS  OutputSizes=1  InputPortWidth=SizeDrv
  Sum : Sum  Inputs=-+|
  Sum1 : Sum  SaturateOnIntegerOverflow=on  InputSameDT=on
  Terminator : Terminator
  Terminator1 : Terminator
  Terminator2 : Terminator
  Turn to yaw : piccolo_library/Flight Mechanics/Turn to yaw  SystemSampleTime=-1
  Yaw Damper : piccolo_library/Controllers/PID Controller  SystemSampleTime=-1  tsamp=tsamp  tdelay=0.25
  Yaw Damper switch : piccolo_library/Logic/Yaw Damper switch  SystemSampleTime=-1
  Actuator : Outport  OutDataType=fixdt(1,16,0)  OutScaling=[]
  wires:
  Mux/1 -> Yaw Damper/4
  Demux/3 -> Mux/3
  Demux/1 -> Mux/1
  Demux/2 -> Terminator2/1
  Scale gains/1 -> Demux/1
  Commands/1 -> Terminator1/1
  Estimates/1 -> Terminator/1
  Selector1/1 -> Yaw Damper/1, Scope/2, Sum/1
  Turn to yaw/1 -> Yaw Damper/2, Scope/1, Sum/2
  Selector8/1 -> Turn to yaw/2
  Selector2/1 -> Turn to yaw/1
  Yaw Damper switch/1 -> Yaw Damper/3
  Selector3/1 -> Yaw Damper switch/2
  Selector17/1 -> Yaw Damper switch/1
  Initial condition/1 -> Mux/2, Yaw Damper/6
  Limits/1 -> Selector6/1
  Settings/1 -> Selector7/1
  Derived/1 -> Selector5/1, Selector8/1, Selector2/1
  Gains/1 -> Selector4/1
  States/1 -> Selector3/1, Selector17/1
  Sensors/1 -> Selector1/1
  Selector4/1 -> Scale gains/1
  Selector5/1 -> Scale gains/2
  Selector6/1 -> Yaw Damper/5, SaturationEx/2
  SaturationEx/1 -> Actuator/1
  Yaw Damper/1 -> Sum1/1
  Selector7/1 -> Sum1/2
  Sum1/1 -> SaturationEx/1
  Sum/1 -> Scope/3

== system HILModelFull/Autopilot/L1 Adaptive Controller LATERAL-DIRECTIONAL/PF Yaw Channel L1 Augmentation ==
  u_psi : Inport
  u2 : Inport  Port=2
  Adaptive Law : Subsystem
  C(s) : Subsystem
  ON : Constant  Value=L1ONOFF
  Product1 : Product  RndMeth=Zero
  State predictor : Subsystem
  Sum1 : Sum  Inputs=-+|
  C_sighat_2 : Outport
  wires:
  Sum1/1 -> Adaptive Law/1(u_psi_tilda)  "u_psi_tilda"
  Adaptive Law/1(sighat_2) -> State predictor/2(sighat_2), C(s)/1(sighat_2)  "sighat_2"
  u_psi/1 -> Sum1/1  "u_psi"
  State predictor/1(u_psi_hat) -> Sum1/2  "u_psi_hat"
  u2/1 -> State predictor/1(u2)
  C(s)/1(C_sighat_2) -> Product1/1
  Product1/1 -> C_sighat_2/1
  ON/1 -> Product1/2

== system HILModelFull/Autopilot/L1 Adaptive Controller LONGITUDINAL/PF Yaw Channel L1 Augmentation ==
  u_psi : Inport
  u2 : Inport  Port=2
  Adaptive Law : Subsystem
  C(s) : Subsystem
  ON : Constant  Value=L1ONOFF
  Product1 : Product  RndMeth=Zero
  State predictor : Subsystem
  Sum1 : Sum  Inputs=-+|
  C_sighat_2 : Outport
  wires:
  ON/1 -> Product1/2
  Product1/1 -> C_sighat_2/1
  C(s)/1(C_sighat_2) -> Product1/1
  u2/1 -> State predictor/1(u2)
  State predictor/1(u_psi_hat) -> Sum1/2  "u_psi_hat"
  u_psi/1 -> Sum1/1  "u_psi"
  Adaptive Law/1(sighat_2) -> C(s)/1(sighat_2), State predictor/2(sighat_2)  "sighat_2"
  Sum1/1 -> Adaptive Law/1(u_psi_tilda)  "u_psi_tilda"

== system HILModelFull/Autopilot/Reshape/ISA Atmosphere Model ==
  height (m) : Inport
  " " : Gain  Gain=20.01  SaturateOnIntegerOverflow=on
  (T/T0)^(g/LR) : Fcn  Expr=u(1)^(ISA_g/(ISA_lapse*ISA_R))
  1/T0 : Gain  Gain=1/ISA_T0  SaturateOnIntegerOverflow=on
  Lapse Rate : Gain  Gain=ISA_lapse  SaturateOnIntegerOverflow=on
  Limit  altitude : Saturate  UpperLimit=ISA_hmax  LowerLimit=0
  P0 : Gain  Gain=ISA_P0  SaturateOnIntegerOverflow=on
  Product : Product  Inputs=*/  SaturateOnIntegerOverflow=on  InputSameDT=on
  Sea Level  Temperature : Constant  Value=ISA_T0
  Sum1 : Sum  Inputs=+-  SaturateOnIntegerOverflow=on  InputSameDT=on
  a : Math  Operator=sqrt  SaturateOnIntegerOverflow=on
  rho0 : Gain  Gain=ISA_rho0  SaturateOnIntegerOverflow=on
  Temperature (K) : Outport  InitialOutput=0
  "Speed of Sound (m/s) " : Outport  Port=2  InitialOutput=0
  "Air Pressure (N/m^2) " : Outport  Port=3  InitialOutput=0
  Air Density (Kg/m^3) : Outport  Port=4  InitialOutput=0
  wires:
  rho0/1 -> Air Density (Kg/m^3)/1
  P0/1 -> "Air Pressure (N/m^2) "/1
  Sea Level  Temperature/1 -> Sum1/1
  Sum1/1 -> a/1, Temperature (K)/1, 1/T0/1
  1/T0/1 -> (T/T0)^(g/LR)/1, Product/2
  (T/T0)^(g/LR)/1 -> P0/1, Product/1
  Product/1 -> rho0/1
  Limit  altitude/1 -> Lapse Rate/1
  height (m)/1 -> Limit  altitude/1
  a/1 -> " "/1
  " "/1 -> "Speed of Sound (m/s) "/1
  Lapse Rate/1 -> Sum1/2

== system HILModelFull/Autopilot/Reshape/ISA Atmosphere Model1 ==
  height (m) : Inport
  " " : Gain  Gain=20.01  SaturateOnIntegerOverflow=on
  (T/T0)^(g/LR) : Fcn  Expr=u(1)^(ISA_g/(ISA_lapse*ISA_R))
  1/T0 : Gain  Gain=1/ISA_T0  SaturateOnIntegerOverflow=on
  Lapse Rate : Gain  Gain=ISA_lapse  SaturateOnIntegerOverflow=on
  Limit  altitude : Saturate  UpperLimit=ISA_hmax  LowerLimit=0
  P0 : Gain  Gain=ISA_P0  SaturateOnIntegerOverflow=on
  Product : Product  Inputs=*/  SaturateOnIntegerOverflow=on  InputSameDT=on
  Sea Level  Temperature : Constant  Value=ISA_T0
  Sum1 : Sum  Inputs=+-  SaturateOnIntegerOverflow=on  InputSameDT=on
  a : Math  Operator=sqrt  SaturateOnIntegerOverflow=on
  rho0 : Gain  Gain=ISA_rho0  SaturateOnIntegerOverflow=on
  Temperature (K) : Outport  InitialOutput=0
  "Speed of Sound (m/s) " : Outport  Port=2  InitialOutput=0
  "Air Pressure (N/m^2) " : Outport  Port=3  InitialOutput=0
  Air Density (Kg/m^3) : Outport  Port=4  InitialOutput=0
  wires:
  rho0/1 -> Air Density (Kg/m^3)/1
  P0/1 -> "Air Pressure (N/m^2) "/1
  Sea Level  Temperature/1 -> Sum1/1
  Sum1/1 -> a/1, Temperature (K)/1, 1/T0/1
  1/T0/1 -> (T/T0)^(g/LR)/1, Product/2
  (T/T0)^(g/LR)/1 -> P0/1, Product/1
  Product/1 -> rho0/1
  Limit  altitude/1 -> Lapse Rate/1
  height (m)/1 -> Limit  altitude/1
  a/1 -> " "/1
  " "/1 -> "Speed of Sound (m/s) "/1
  Lapse Rate/1 -> Sum1/2

== system HILModelFull/Autopilot/Reshape/ISA Atmosphere Model2 ==
  height (m) : Inport
  " " : Gain  Gain=20.01  SaturateOnIntegerOverflow=on
  (T/T0)^(g/LR) : Fcn  Expr=u(1)^(ISA_g/(ISA_lapse*ISA_R))
  1/T0 : Gain  Gain=1/ISA_T0  SaturateOnIntegerOverflow=on
  Lapse Rate : Gain  Gain=ISA_lapse  SaturateOnIntegerOverflow=on
  Limit  altitude : Saturate  UpperLimit=ISA_hmax  LowerLimit=0
  P0 : Gain  Gain=ISA_P0  SaturateOnIntegerOverflow=on
  Product : Product  Inputs=*/  SaturateOnIntegerOverflow=on  InputSameDT=on
  Sea Level  Temperature : Constant  Value=ISA_T0
  Sum1 : Sum  Inputs=+-  SaturateOnIntegerOverflow=on  InputSameDT=on
  a : Math  Operator=sqrt  SaturateOnIntegerOverflow=on
  rho0 : Gain  Gain=ISA_rho0  SaturateOnIntegerOverflow=on
  Temperature (K) : Outport  InitialOutput=0
  "Speed of Sound (m/s) " : Outport  Port=2  InitialOutput=0
  "Air Pressure (N/m^2) " : Outport  Port=3  InitialOutput=0
  Air Density (Kg/m^3) : Outport  Port=4  InitialOutput=0
  wires:
  rho0/1 -> Air Density (Kg/m^3)/1
  P0/1 -> "Air Pressure (N/m^2) "/1
  Sea Level  Temperature/1 -> Sum1/1
  Sum1/1 -> a/1, Temperature (K)/1, 1/T0/1
  1/T0/1 -> (T/T0)^(g/LR)/1, Product/2
  (T/T0)^(g/LR)/1 -> P0/1, Product/1
  Product/1 -> rho0/1
  Limit  altitude/1 -> Lapse Rate/1
  height (m)/1 -> Limit  altitude/1
  a/1 -> " "/1
  " "/1 -> "Speed of Sound (m/s) "/1
  Lapse Rate/1 -> Sum1/2

== system HILModelFull/Autopilot/Reshape/Subsystem ==
  "XYZ, ltp" : Inport  OutDataType=fixdt(1,16,0)  OutScaling=[]
  Href : Inport  Port=2  OutDataType=fixdt(1,16,0)  OutScaling=[]
  Flat Earth to LLA : aerolibtransform2/Flat Earth to LLA  SystemSampleTime=-1  units=Metric (MKS)  ptype=Earth (WGS84)  F=1/298.257223563  R=6378137  LL0=[35 -120]  psi=0
  "LL, deg" : Outport  OutDataType=fixdt(1,16,0)  OutScaling=[]
  "A, m" : Outport  Port=2  OutDataType=fixdt(1,16,0)  OutScaling=[]
  wires:
  Flat Earth to LLA/1 -> "LL, deg"/1
  Flat Earth to LLA/2 -> "A, m"/1
  "XYZ, ltp"/1 -> Flat Earth to LLA/1
  Href/1 -> Flat Earth to LLA/2

== system HILModelFull/Autopilot/Reshape/norm ==
  In1 : Inport  OutDataType=fixdt(1,16,0)  OutScaling=[]
  Math Function : Math  Operator=sqrt  SaturateOnIntegerOverflow=on
  dot : aerolibasang/Dynamic Pressure/dot  SystemSampleTime=-1
  Out1 : Outport  OutDataType=fixdt(1,16,0)  OutScaling=[]
  wires:
  dot/1 -> Math Function/1
  Math Function/1 -> Out1/1
  In1/1 -> dot/1

== system HILModelFull/Plant Model/Generic Sensor/Dynamics ==
  "Sens " : Inport
  Constant : Constant  Value=dtype_g
  No Dynamics : Subsystem
  Second-order Dynamics : Subsystem  AncestorBlock=aerolibnav/Three-axis Accelerometer/Dynamics/If Action Subsystem
  Switch : Switch  Threshold=0.5
  Sens Dyn : Outport
  wires:
  "Sens "/1 -> Second-order Dynamics/1(In1), No Dynamics/1(In1)
  No Dynamics/1(Out1) -> Switch/3
  Second-order Dynamics/1(Out1) -> Switch/1
  Switch/1 -> Sens Dyn/1
  Constant/1 -> Switch/2

== system HILModelFull/Plant Model/Plant/6-DOF EOM ==
  "[F,M]" : Inport
  Vb Corr : Inport  Orientation=left  Port=2
  Angular Rates : Integrator  InitialCondition=PQR_0'  LimitOutput=on  UpperSaturationLimit=10  LowerSaturationLimit=-10
  Demux1 : Demux  Outputs=[3 3]
  Euler Angles : Integrator  InitialCondition=Euler_0'
  Get Euler Dot : Subsystem
      mask Display:
      | port_label('input', 1, 'p, q, r')
      | port_label('input', 2, 'Euler')
      | port_label('output', 1, 'Euler_dot')
  Mux : Mux  Orientation=left  Inputs=[3;3]
  NED2NEU : Gain  Gain=[1 0 0;0 1 0;0 0 -1]  Multiplication=Matrix(K*u)  SaturateOnIntegerOverflow=on
  Position : Integrator  InitialCondition=Pos_0'
  RB2L * Vb : Product  Multiplication=Matrix(*)  SaturateOnIntegerOverflow=on  InputSameDT=on
  RB2LTP : Subsystem
  Velocities Body : Integrator  InitialCondition=Vb_0'  LimitOutput=on  UpperSaturationLimit=200  LowerSaturationLimit=-200
  "[V1,2,3,W1,2,3]" : Subsystem
  X,Y,Z (LTP) : Outport
  "Vx, Vy, Vz" : Outport  Port=2
  Euler : Outport  Port=3
  "p, q, r" : Outport  Orientation=left  Port=4
  Vb : Outport  Port=5
  Ab meas : Outport  Port=6
  wires:
  "[V1,2,3,W1,2,3]"/1("Acc_meas ") -> Ab meas/1
  Euler Angles/1 -> Euler/1, "[V1,2,3,W1,2,3]"/2(Euler), Get Euler Dot/2(Euler), RB2LTP/1(Euler)
  Demux1/1 -> Velocities Body/1
  "[V1,2,3,W1,2,3]"/2(V*dot) -> Demux1/1
  Demux1/2 -> Angular Rates/1
  "[F,M]"/1 -> "[V1,2,3,W1,2,3]"/1("[F ; M]")
  RB2LTP/1(Rot) -> RB2L * Vb/1
  Velocities Body/1 -> Vb/1, RB2L * Vb/2
  Mux/1 -> "[V1,2,3,W1,2,3]"/3(V*)
  Position/1 -> X,Y,Z (LTP)/1
  Angular Rates/1 -> Get Euler Dot/1(p,q,r), "p, q, r"/1, Mux/2
  RB2L * Vb/1 -> NED2NEU/1, "Vx, Vy, Vz"/1  "NED"
  NED2NEU/1 -> Position/1
  Get Euler Dot/1(Euler_dot) -> Euler Angles/1
  Vb Corr/1 -> Mux/1

== system HILModelFull/Plant Model/Plant/Engine Model ==
  dt : Inport
  Vmag : Inport  Port=2
  Constant4 : Constant  Value=0
  Get To1 : Subsystem
  Mux : Mux  Inputs=2
  Mux1 : Mux  Inputs=3
  Thrust Available (lbs) : Fcn  Expr=u(1) - 0.047*sqrt(u(1))*u(2)
  kg2N : Gain  Gain=ISA_g  SaturateOnIntegerOverflow=on
  lbs2kg : Gain  Gain=0.45359237  SaturateOnIntegerOverflow=on
  Thrust : Outport
  wires:
  dt/1 -> Get To1/1(dt)
  Get To1/1(To) -> Mux/1
  Mux/1 -> Thrust Available (lbs)/1
  Thrust Available (lbs)/1 -> lbs2kg/1
  Vmag/1 -> Mux/2
  Mux1/1 -> Thrust/1
  lbs2kg/1 -> kg2N/1
  Constant4/1 -> Mux1/2, Mux1/3
  kg2N/1 -> Mux1/1

== system HILModelFull/Plant Model/Plant/Forces and Moments ==
  Wind e : Inport
  Rho : Inport  Port=2
  "de, deg" : Inport  Port=3
  da,deg : Inport  Port=4
  "dr, deg" : Inport  Port=5
  "df, deg" : Inport  Port=6
  "Vx, Vy, Vz " : Inport  Port=7
  Euler : Inport  Port=8  PortDimensions=3
  p,q,r : Inport  Port=9
  Alpha/Beta : Subsystem
  Body Frame F & M : Subsystem
  Get Grav Force in Body : Subsystem
  Gravitational Force : Constant  Value=[0 0 mass*ISA_g]  VectorParams1D=off
  Mux1 : Mux  Inputs=2
  NED(u)2b : Subsystem
  Scope : Scope
      settings: SaveName=ScopeData5
  Selector : Selector  IndexOptions=Index vector (dialog)  Indices=3  OutputSizes=1  InputPortWidth=3
  Selector1 : Selector  Orientation=up  IndexOptions=Index vector (dialog)  Indices=3  OutputSizes=1  InputPortWidth=3
  Sum : Sum  Inputs=|++  SaturateOnIntegerOverflow=on
  Vair : Sum  Inputs=+-  SaturateOnIntegerOverflow=on  InputSameDT=on
  Airspeed : Outport
  Forces : Outport  Port=2
  Moments : Outport  Port=3
  Vb Corr : Outport  Port=4
  q : Outport  Port=5
  wires:
  Get Grav Force in Body/1(Grav Force (Body)) -> Sum/2
  Selector1/1 -> Mux1/2
  Mux1/1 -> Scope/1
  Selector/1 -> Mux1/1
  Alpha/Beta/5(q) -> q/1
  "Vx, Vy, Vz "/1 -> Vair/1
  Vair/1 -> NED(u)2b/1(V w)
  Euler/1 -> NED(u)2b/2(Euler), Get Grav Force in Body/1(Euler)
  Rho/1 -> Alpha/Beta/2(Rho)
  NED(u)2b/1(Vb Corr) -> Alpha/Beta/1("Vx, Vy, Vz (Body)"), Vb Corr/1
  Body Frame F & M/2(M_b) -> Moments/1
  Gravitational Force/1 -> Get Grav Force in Body/2(Grav Force)
  Body Frame F & M/1(F_b) -> Selector/1, Sum/1
  Sum/1 -> Selector1/1, Forces/1
  Alpha/Beta/3(qS) -> Body Frame F & M/3(qs)
  Alpha/Beta/4(Speed) -> Body Frame F & M/4(Airspeed), Airspeed/1
  "df, deg"/1 -> Body Frame F & M/8("df, deg")
  p,q,r/1 -> Body Frame F & M/9(p,q,r)
  Alpha/Beta/2("beta, deg") -> Body Frame F & M/2("Beta, deg")
  "dr, deg"/1 -> Body Frame F & M/7("dr, deg")
  da,deg/1 -> Body Frame F & M/6("da, deg")
  Alpha/Beta/1("alpha, deg") -> Body Frame F & M/1("Alpha, deg")
  "de, deg"/1 -> Body Frame F & M/5("de, deg")
  Wind e/1 -> Vair/2
